simulink model "AW_PMSMwTorqueRipple"  (R2021b)
settings: Solver=VariableStepAuto  StartTime=0.0  StopTime=100  MaxStep=ts  RelTol=1e-3
values from neighbouring files (symbols this model uses):
  alfa = atan(sqrt(3)*dia / (dia + 2*dib))    [AW_RippleModel_InitFcn.m]
  delta_T = diqA*K_t    [AW_RippleModel_InitFcn.m]
  Jz = 0.753    [AW_RippleModel_InitFcn.m]
  K_t = 17.5    [AW_RippleModel_InitFcn.m]
  p = 24    [AW_RippleModel_InitFcn.m]
  PID_GA_b = 1    [AW_RippleModel_InitFcn.m]
  PID_GA_Kd = 4.772*(88.300/1000)    (= 0.4213676)    [AW_RippleModel_InitFcn.m]
  PID_GA_Ki = 4.772/(0.153/1000)    (= 31189.5424837)    [AW_RippleModel_InitFcn.m]
  PID_GA_Kp = 4.772    [AW_RippleModel_InitFcn.m]
  PID_Ki = Jz  * ((2*pi*fref)^2)    (= 2972.72484561)    [AW_RippleModel_InitFcn.m]
  PID_Kp = (2*eref*Jz) * (2*pi*fref)    (= 85.1622936535)    [AW_RippleModel_InitFcn.m]
  Tn = 50    [AW_RippleModel_InitFcn.m]
libraries: slpidlib x7, cstblocks x4, simulink x1, fuzblock x1
settings Model: Creator=AW  LastModifiedBy=adria
settings SolverCC: AlgebraicLoopSolver=TrustRegion  PositivePriorityOrder=on
settings DataIOCC: ReturnWorkspaceOutputs=off
settings DebuggingCC: SFMachineParentedDataDiag=warning  ArithmeticOperatorsInVariantConditions=warning
settings SFSimCC: SimUseLocalCustomCode=off  CustomCodeUndefinedFunction=UseInterfaceOnly
settings RTWCC: RTWUseLocalCustomCode=off

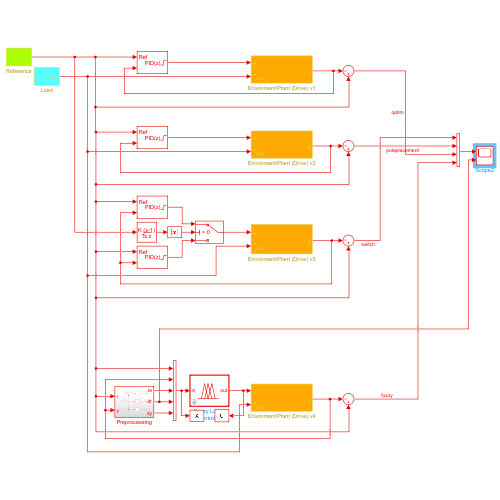
[thumbnail: Simulink's stored preview of the top-level diagram]
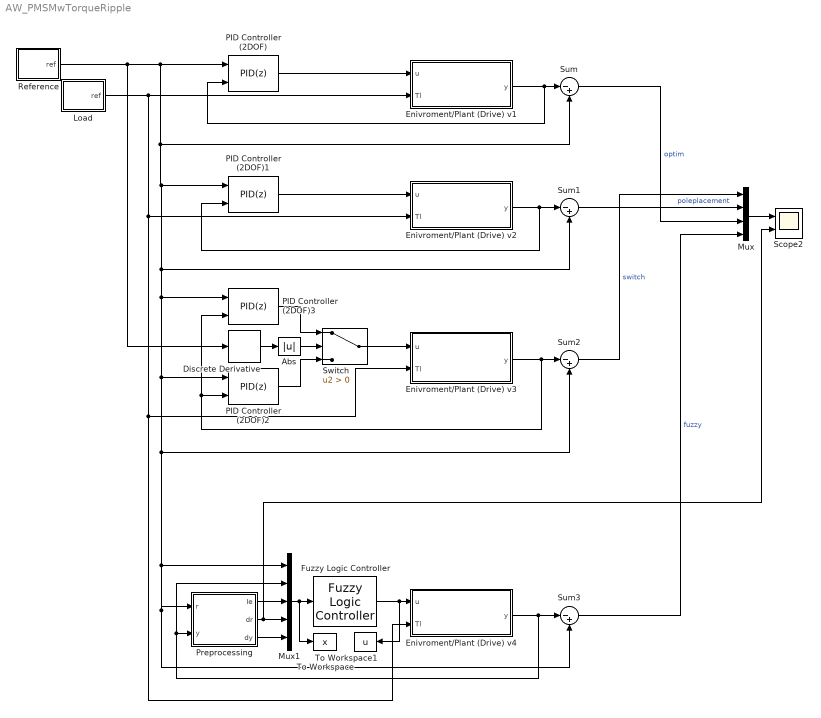
== system AW_PMSMwTorqueRipple ==
  Abs : Abs
  Discrete Derivative : simulink/Quick Insert/Discrete/Discrete Derivative  gainval=1.0  ICPrevScaledInput=0.0  OutMin=[]  OutMax=[]  OutDataType=fixdt(1, 16)  OutScaling=2^-10  DoSatur=off
      settings: SourceProductBaseCode=SL
  Enivroment/Plant (Drive) v1 : Subsystem
      mask Display:
      | port_label('input', 1, 'u', 'texmode', 'on')
      | port_label('input', 2, 'T_{load}', 'texmode', 'on')
      | port_label('output', 1, 'y', 'texmode', 'on')
  Enivroment/Plant (Drive) v2 : Subsystem
      mask Display:
      | port_label('input', 1, 'u', 'texmode', 'on')
      | port_label('input', 2, 'T_{load}', 'texmode', 'on')
      | port_label('output', 1, 'y', 'texmode', 'on')
  Enivroment/Plant (Drive) v3 : Subsystem
      mask Display:
      | port_label('input', 1, 'u', 'texmode', 'on')
      | port_label('input', 2, 'T_{load}', 'texmode', 'on')
      | port_label('output', 1, 'y', 'texmode', 'on')
  Enivroment/Plant (Drive) v4 : Subsystem
      mask Display:
      | port_label('input', 1, 'u', 'texmode', 'on')
      | port_label('input', 2, 'T_{load}', 'texmode', 'on')
      | port_label('output', 1, 'y', 'texmode', 'on')
  Fuzzy Logic Controller : fuzblock/Fuzzy Logic  Controller  FIS=PMSM_SpeedController  OutputSampleNumber=101  DataType=double  FuzzifiedInputs=off  RuleFiringStrengths=off  RuleOutputs=off  AggregatedOutputs=off  SimulateUsing=Code generation  OutOfRangeInputValueMessage=warning  NoRuleFiredMessage=warning  EmptyOutputFuzzySetMessage=warning
  Load : Subsystem
      mask Display: port_label('output', 1, 'T_{load}', 'texmode', 'on')
  Mux : Mux
  Mux1 : Mux  Inputs=5
  PID Controller (2DOF) : slpidlib/PID Controller (2DOF)  Controller=PID  Form=Parallel  TimeDomain=Discrete-time  UseExternalTs=off  SampleTime=-1  IntegratorMethod=Forward Euler  FilterMethod=Forward Euler  ControllerParametersSource=internal  P=PID_GA_Kp  I=PID_GA_Ki  D=PID_GA_Kd  UseFilter=on  N=100  b=PID_GA_b  c=PID_GA_c  TunerSelectOption=Transfer Function Based (PID Tuner App)  InitialConditionSource=internal  InitialConditionForIntegrator=0  InitialConditionForFilter=0  DifferentiatorICPrevScaledInput=0  ExternalReset=none  TrackingMode=off  Kt=1  LimitOutput=on  SatLimitsSource=internal  UpperSaturationLimit=6  LowerSaturationLimit=-6  LinearizeAsGain=on  AntiWindupMode=none  Kb=1  POutMin=[]  POutMax=[]  IOutMin=[]  IOutMax=[]  DOutMin=[]  DOutMax=[]  NOutMin=[]  NOutMax=[]  bOutMin=[]  bOutMax=[]  cOutMin=[]  cOutMax=[]  SumOutMin=[]  SumOutMax=[]  SaturationOutMin=[]  SaturationOutMax=[]  PParamMin=[]  PParamMax=[]  IParamMin=[]  IParamMax=[]  DParamMin=[]  DParamMax=[]  NParamMin=[]  NParamMax=[]  bParamMin=[]  bParamMax=[]  cParamMin=[]  cParamMax=[]  KbParamMin=[]  KbParamMax=[]  KtParamMin=[]  KtParamMax=[]  KbOutMin=[]  KbOutMax=[]  KtOutMin=[]  KtOutMax=[]  IntegratorOutMin=[]  IntegratorOutMax=[]  FilterOutMin=[]  FilterOutMax=[]  SumI1OutMin=[]  SumI1OutMax=[]  SumI2OutMin=[]  SumI2OutMax=[]  SumI3OutMin=[]  SumI3OutMax=[]  SumI4OutMin=[]  SumI4OutMax=[]  SumDOutMin=[]  SumDOutMax=[]  Sum1OutMin=[]  Sum1OutMax=[]  Sum2OutMin=[]  Sum2OutMax=[]  Sum3OutMin=[]  Sum3OutMax=[]  DifferentiatorOutMin=[]  DifferentiatorOutMax=[]  FilterDiffOutCoefMin=[]  FilterDiffOutCoefMax=[]  ReciprocalOutMin=[]  ReciprocalOutMax=[]  SumDenOutMin=[]  SumDenOutMax=[]  SumNumOutMin=[]  SumNumOutMax=[]  DivideOutMin=[]  DivideOutMax=[]  UdiffTsProdOutMin=[]  UdiffTsProdOutMax=[]  NTsProdOutMin=[]  NTsProdOutMax=[]  UintegralTsProdOutMin=[]  UintegralTsProdOutMax=[]  UngainTsProdOutMin=[]  UngainTsProdOutMax=[]  IntegratorContinuousStateAttributes=''  IntegratorStateMustResolveToSignalObject=off  IntegratorRTWStateStorageClass=Auto  FilterContinuousStateAttributes=''  FilterStateMustResolveToSignalObject=off  FilterRTWStateStorageClass=Auto  ParallelPVariant=InternalParameters  IdealPVariant=Disabled  IVariant=InternalParameters  DVariant=InternalParameters  bVariant=InternalParameters  cVariant=InternalParameters  IntegratorVariant=Discrete  SatVariant=Enabled  AWVariant=Passthrough  PCopyVariant=Disabled  TRVariant=Disabled  FdbkBlocksVariant=Forward  IdealPFdbkVariant=Disabled  SatFdbkVariant=Disabled  DerivativeFilterVariant=ForwardEulerFilter  NVariant=InternalParameters  NCopyVariant=Disabled  FilterICVariant=InternalICsFilter  IntegratorICVariant=InternalICs  ExternalResetVariant=Disabled  TRSumVariant=Passthrough  SumFdbkVariant=Disabled  SumVariant=Sum_PID  TsampFilterVariant=InternalTs  TsampNgainVariant=Passthrough  TsampIntegralVariant=Passthrough  ExternalSaturationOutDataTypeStr=Inherit: Same as second input
      settings: SourceProductBaseCode=SL
  PID Controller (2DOF)1 : slpidlib/PID Controller (2DOF)  Controller=PID  Form=Parallel  TimeDomain=Discrete-time  UseExternalTs=off  SampleTime=-1  IntegratorMethod=Forward Euler  FilterMethod=Forward Euler  ControllerParametersSource=internal  P=PID_Kp  I=PID_Ki  D=0  UseFilter=on  N=100  b=1  c=0  TunerSelectOption=Transfer Function Based (PID Tuner App)  InitialConditionSource=internal  InitialConditionForIntegrator=0  InitialConditionForFilter=0  DifferentiatorICPrevScaledInput=0  ExternalReset=none  TrackingMode=off  Kt=1  LimitOutput=on  SatLimitsSource=internal  UpperSaturationLimit=6  LowerSaturationLimit=-6  LinearizeAsGain=on  AntiWindupMode=none  Kb=1  POutMin=[]  POutMax=[]  IOutMin=[]  IOutMax=[]  DOutMin=[]  DOutMax=[]  NOutMin=[]  NOutMax=[]  bOutMin=[]  bOutMax=[]  cOutMin=[]  cOutMax=[]  SumOutMin=[]  SumOutMax=[]  SaturationOutMin=[]  SaturationOutMax=[]  PParamMin=[]  PParamMax=[]  IParamMin=[]  IParamMax=[]  DParamMin=[]  DParamMax=[]  NParamMin=[]  NParamMax=[]  bParamMin=[]  bParamMax=[]  cParamMin=[]  cParamMax=[]  KbParamMin=[]  KbParamMax=[]  KtParamMin=[]  KtParamMax=[]  KbOutMin=[]  KbOutMax=[]  KtOutMin=[]  KtOutMax=[]  IntegratorOutMin=[]  IntegratorOutMax=[]  FilterOutMin=[]  FilterOutMax=[]  SumI1OutMin=[]  SumI1OutMax=[]  SumI2OutMin=[]  SumI2OutMax=[]  SumI3OutMin=[]  SumI3OutMax=[]  SumI4OutMin=[]  SumI4OutMax=[]  SumDOutMin=[]  SumDOutMax=[]  Sum1OutMin=[]  Sum1OutMax=[]  Sum2OutMin=[]  Sum2OutMax=[]  Sum3OutMin=[]  Sum3OutMax=[]  DifferentiatorOutMin=[]  DifferentiatorOutMax=[]  FilterDiffOutCoefMin=[]  FilterDiffOutCoefMax=[]  ReciprocalOutMin=[]  ReciprocalOutMax=[]  SumDenOutMin=[]  SumDenOutMax=[]  SumNumOutMin=[]  SumNumOutMax=[]  DivideOutMin=[]  DivideOutMax=[]  UdiffTsProdOutMin=[]  UdiffTsProdOutMax=[]  NTsProdOutMin=[]  NTsProdOutMax=[]  UintegralTsProdOutMin=[]  UintegralTsProdOutMax=[]  UngainTsProdOutMin=[]  UngainTsProdOutMax=[]  IntegratorContinuousStateAttributes=''  IntegratorStateMustResolveToSignalObject=off  IntegratorRTWStateStorageClass=Auto  FilterContinuousStateAttributes=''  FilterStateMustResolveToSignalObject=off  FilterRTWStateStorageClass=Auto  ParallelPVariant=InternalParameters  IdealPVariant=Disabled  IVariant=InternalParameters  DVariant=InternalParameters  bVariant=InternalParameters  cVariant=InternalParameters  IntegratorVariant=Discrete  SatVariant=Enabled  AWVariant=Passthrough  PCopyVariant=Disabled  TRVariant=Disabled  FdbkBlocksVariant=Forward  IdealPFdbkVariant=Disabled  SatFdbkVariant=Disabled  DerivativeFilterVariant=ForwardEulerFilter  NVariant=InternalParameters  NCopyVariant=Disabled  FilterICVariant=InternalICsFilter  IntegratorICVariant=InternalICs  ExternalResetVariant=Disabled  TRSumVariant=Passthrough  SumFdbkVariant=Disabled  SumVariant=Sum_PID  TsampFilterVariant=InternalTs  TsampNgainVariant=Passthrough  TsampIntegralVariant=Passthrough  ExternalSaturationOutDataTypeStr=Inherit: Same as second input
      settings: SourceProductBaseCode=SL
  PID Controller (2DOF)2 : slpidlib/PID Controller (2DOF)  Controller=PID  Form=Parallel  TimeDomain=Discrete-time  UseExternalTs=off  SampleTime=-1  IntegratorMethod=Forward Euler  FilterMethod=Forward Euler  ControllerParametersSource=internal  P=4.772  I=4.772/(0.153/1000)  D=4.772*(88.300/1000)  UseFilter=on  N=100  b=1  c=0.258  TunerSelectOption=Transfer Function Based (PID Tuner App)  InitialConditionSource=internal  InitialConditionForIntegrator=0  InitialConditionForFilter=0  DifferentiatorICPrevScaledInput=0  ExternalReset=none  TrackingMode=off  Kt=1  LimitOutput=on  SatLimitsSource=internal  UpperSaturationLimit=6  LowerSaturationLimit=-6  LinearizeAsGain=on  AntiWindupMode=none  Kb=1  POutMin=[]  POutMax=[]  IOutMin=[]  IOutMax=[]  DOutMin=[]  DOutMax=[]  NOutMin=[]  NOutMax=[]  bOutMin=[]  bOutMax=[]  cOutMin=[]  cOutMax=[]  SumOutMin=[]  SumOutMax=[]  SaturationOutMin=[]  SaturationOutMax=[]  PParamMin=[]  PParamMax=[]  IParamMin=[]  IParamMax=[]  DParamMin=[]  DParamMax=[]  NParamMin=[]  NParamMax=[]  bParamMin=[]  bParamMax=[]  cParamMin=[]  cParamMax=[]  KbParamMin=[]  KbParamMax=[]  KtParamMin=[]  KtParamMax=[]  KbOutMin=[]  KbOutMax=[]  KtOutMin=[]  KtOutMax=[]  IntegratorOutMin=[]  IntegratorOutMax=[]  FilterOutMin=[]  FilterOutMax=[]  SumI1OutMin=[]  SumI1OutMax=[]  SumI2OutMin=[]  SumI2OutMax=[]  SumI3OutMin=[]  SumI3OutMax=[]  SumI4OutMin=[]  SumI4OutMax=[]  SumDOutMin=[]  SumDOutMax=[]  Sum1OutMin=[]  Sum1OutMax=[]  Sum2OutMin=[]  Sum2OutMax=[]  Sum3OutMin=[]  Sum3OutMax=[]  DifferentiatorOutMin=[]  DifferentiatorOutMax=[]  FilterDiffOutCoefMin=[]  FilterDiffOutCoefMax=[]  ReciprocalOutMin=[]  ReciprocalOutMax=[]  SumDenOutMin=[]  SumDenOutMax=[]  SumNumOutMin=[]  SumNumOutMax=[]  DivideOutMin=[]  DivideOutMax=[]  UdiffTsProdOutMin=[]  UdiffTsProdOutMax=[]  NTsProdOutMin=[]  NTsProdOutMax=[]  UintegralTsProdOutMin=[]  UintegralTsProdOutMax=[]  UngainTsProdOutMin=[]  UngainTsProdOutMax=[]  IntegratorContinuousStateAttributes=''  IntegratorStateMustResolveToSignalObject=off  IntegratorRTWStateStorageClass=Auto  FilterContinuousStateAttributes=''  FilterStateMustResolveToSignalObject=off  FilterRTWStateStorageClass=Auto  ParallelPVariant=InternalParameters  IdealPVariant=Disabled  IVariant=InternalParameters  DVariant=InternalParameters  bVariant=InternalParameters  cVariant=InternalParameters  IntegratorVariant=Discrete  SatVariant=Enabled  AWVariant=Passthrough  PCopyVariant=Disabled  TRVariant=Disabled  FdbkBlocksVariant=Forward  IdealPFdbkVariant=Disabled  SatFdbkVariant=Disabled  DerivativeFilterVariant=ForwardEulerFilter  NVariant=InternalParameters  NCopyVariant=Disabled  FilterICVariant=InternalICsFilter  IntegratorICVariant=InternalICs  ExternalResetVariant=Disabled  TRSumVariant=Passthrough  SumFdbkVariant=Disabled  SumVariant=Sum_PID  TsampFilterVariant=InternalTs  TsampNgainVariant=Passthrough  TsampIntegralVariant=Passthrough  ExternalSaturationOutDataTypeStr=Inherit: Same as second input
      settings: SourceProductBaseCode=SL
  PID Controller (2DOF)3 : slpidlib/PID Controller (2DOF)  Controller=PID  Form=Parallel  TimeDomain=Discrete-time  UseExternalTs=off  SampleTime=-1  IntegratorMethod=Forward Euler  FilterMethod=Forward Euler  ControllerParametersSource=internal  P=PID_Kp  I=PID_Ki  D=0  UseFilter=on  N=100  b=1  c=0  TunerSelectOption=Transfer Function Based (PID Tuner App)  InitialConditionSource=internal  InitialConditionForIntegrator=0  InitialConditionForFilter=0  DifferentiatorICPrevScaledInput=0  ExternalReset=none  TrackingMode=off  Kt=1  LimitOutput=on  SatLimitsSource=internal  UpperSaturationLimit=6  LowerSaturationLimit=-6  LinearizeAsGain=on  AntiWindupMode=none  Kb=1  POutMin=[]  POutMax=[]  IOutMin=[]  IOutMax=[]  DOutMin=[]  DOutMax=[]  NOutMin=[]  NOutMax=[]  bOutMin=[]  bOutMax=[]  cOutMin=[]  cOutMax=[]  SumOutMin=[]  SumOutMax=[]  SaturationOutMin=[]  SaturationOutMax=[]  PParamMin=[]  PParamMax=[]  IParamMin=[]  IParamMax=[]  DParamMin=[]  DParamMax=[]  NParamMin=[]  NParamMax=[]  bParamMin=[]  bParamMax=[]  cParamMin=[]  cParamMax=[]  KbParamMin=[]  KbParamMax=[]  KtParamMin=[]  KtParamMax=[]  KbOutMin=[]  KbOutMax=[]  KtOutMin=[]  KtOutMax=[]  IntegratorOutMin=[]  IntegratorOutMax=[]  FilterOutMin=[]  FilterOutMax=[]  SumI1OutMin=[]  SumI1OutMax=[]  SumI2OutMin=[]  SumI2OutMax=[]  SumI3OutMin=[]  SumI3OutMax=[]  SumI4OutMin=[]  SumI4OutMax=[]  SumDOutMin=[]  SumDOutMax=[]  Sum1OutMin=[]  Sum1OutMax=[]  Sum2OutMin=[]  Sum2OutMax=[]  Sum3OutMin=[]  Sum3OutMax=[]  DifferentiatorOutMin=[]  DifferentiatorOutMax=[]  FilterDiffOutCoefMin=[]  FilterDiffOutCoefMax=[]  ReciprocalOutMin=[]  ReciprocalOutMax=[]  SumDenOutMin=[]  SumDenOutMax=[]  SumNumOutMin=[]  SumNumOutMax=[]  DivideOutMin=[]  DivideOutMax=[]  UdiffTsProdOutMin=[]  UdiffTsProdOutMax=[]  NTsProdOutMin=[]  NTsProdOutMax=[]  UintegralTsProdOutMin=[]  UintegralTsProdOutMax=[]  UngainTsProdOutMin=[]  UngainTsProdOutMax=[]  IntegratorContinuousStateAttributes=''  IntegratorStateMustResolveToSignalObject=off  IntegratorRTWStateStorageClass=Auto  FilterContinuousStateAttributes=''  FilterStateMustResolveToSignalObject=off  FilterRTWStateStorageClass=Auto  ParallelPVariant=InternalParameters  IdealPVariant=Disabled  IVariant=InternalParameters  DVariant=InternalParameters  bVariant=InternalParameters  cVariant=InternalParameters  IntegratorVariant=Discrete  SatVariant=Enabled  AWVariant=Passthrough  PCopyVariant=Disabled  TRVariant=Disabled  FdbkBlocksVariant=Forward  IdealPFdbkVariant=Disabled  SatFdbkVariant=Disabled  DerivativeFilterVariant=ForwardEulerFilter  NVariant=InternalParameters  NCopyVariant=Disabled  FilterICVariant=InternalICsFilter  IntegratorICVariant=InternalICs  ExternalResetVariant=Disabled  TRSumVariant=Passthrough  SumFdbkVariant=Disabled  SumVariant=Sum_PID  TsampFilterVariant=InternalTs  TsampNgainVariant=Passthrough  TsampIntegralVariant=Passthrough  ExternalSaturationOutDataTypeStr=Inherit: Same as second input
      settings: SourceProductBaseCode=SL
  Preprocessing : Subsystem
  Reference : Subsystem
      mask Display: port_label('output', 1, 'y_{ref}', 'texmode', 'on')
  Scope2 : Scope  NumInputPorts=2
  Sum{,1..3} (4 alike) : Sum  Inputs=|-+
  Switch : Switch  Criteria=u2 > Threshold
  To Workspace : ToWorkspace  VariableName=x  SaveFormat=Timeseries  SampleTime=-1
  To Workspace1 : ToWorkspace  VariableName=u  SaveFormat=Timeseries  SampleTime=-1
  wires:
  Sum/1 -> Mux/3  "optim"
  Sum1/1 -> Mux/2  "poleplacement"
  Load/1(ref) -> Enivroment/Plant (Drive) v2/2(Tl), Enivroment/Plant (Drive) v4/2(Tl), Enivroment/Plant (Drive) v3/2(Tl), Enivroment/Plant (Drive) v1/2(Tl)
  Enivroment/Plant (Drive) v2/1(y) -> Sum1/1, PID Controller (2DOF)1/2
  PID Controller (2DOF)1/1 -> Enivroment/Plant (Drive) v2/1(u)
  Mux/1 -> Scope2/1
  Discrete Derivative/1 -> Abs/1
  Abs/1 -> Switch/2
  PID Controller (2DOF)3/1 -> Switch/1
  Switch/1 -> Enivroment/Plant (Drive) v3/1(u)
  Enivroment/Plant (Drive) v3/1(y) -> Sum2/1, PID Controller (2DOF)3/2, PID Controller (2DOF)2/2
  Sum2/1 -> Mux/1  "switch"
  PID Controller (2DOF)2/1 -> Switch/3
  Preprocessing/3(dy) -> Mux1/5
  Preprocessing/2(dr) -> Scope2/2, Mux1/4
  Preprocessing/1(Ie) -> Mux1/3
  Mux1/1 -> To Workspace/1, Fuzzy Logic Controller/1
  Fuzzy Logic Controller/1 -> To Workspace1/1, Enivroment/Plant (Drive) v4/1(u)
  Enivroment/Plant (Drive) v4/1(y) -> Sum3/1, Preprocessing/2(y), Mux1/2
  PID Controller (2DOF)/1 -> Enivroment/Plant (Drive) v1/1(u)
  Sum3/1 -> Mux/4  "fuzzy"
  Enivroment/Plant (Drive) v1/1(y) -> Sum/1, PID Controller (2DOF)/2
  Reference/1(ref) -> Discrete Derivative/1, Sum/2, Sum1/2, Sum2/2, Mux1/1, Preprocessing/1(r), Sum3/2, PID Controller (2DOF)2/1, PID Controller (2DOF)3/1, PID Controller (2DOF)1/1, PID Controller (2DOF)/1

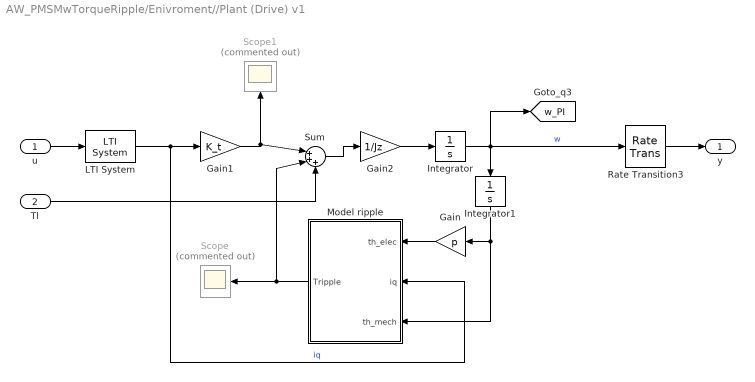
== system AW_PMSMwTorqueRipple/Enivroment//Plant (Drive) v1 ==
  u : Inport
  Tl : Inport  Port=2
  Gain : Gain  Gain=p
  Gain1 : Gain  Gain=K_t
  Gain2 : Gain  Gain=1/Jz
  Integrator : Integrator
  Integrator1 : Integrator
  LTI System : cstblocks/LTI System  sys=h_curr  IC=[]
  Model ripple : Subsystem
  Rate Transition3 : RateTransition  OutPortSampleTime=ts
  Scope : Scope  Commented=on
  Scope1 : Scope  Commented=on
  Sum : Sum  Inputs=|+++
  y : Outport  VectorParamsAs1DForOutWhenUnconnected=off
  tag scope: w_PI=global
  wires:
  Gain/1 -> Model ripple/1(th_elec)
  Integrator/1 -> [w_PI], Rate Transition3/1, Integrator1/1  "w"
  u/1 -> LTI System/1
  Gain2/1 -> Integrator/1
  Sum/1 -> Gain2/1
  Model ripple/1(Tripple) -> Sum/2, Scope/1
  Gain1/1 -> Scope1/1, Sum/1
  Integrator1/1 -> Model ripple/3(th_mech), Gain/1
  LTI System/1 -> Gain1/1, Model ripple/2(iq)  "iq"
  Tl/1 -> Sum/3
  Rate Transition3/1 -> y/1

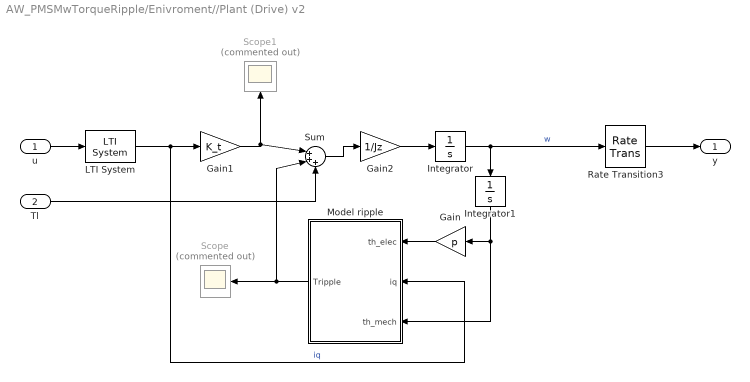
== system AW_PMSMwTorqueRipple/Enivroment//Plant (Drive) v2 ==
  u : Inport
  Tl : Inport  Port=2
  Gain : Gain  Gain=p
  Gain1 : Gain  Gain=K_t
  Gain2 : Gain  Gain=1/Jz
  Integrator : Integrator
  Integrator1 : Integrator
  LTI System : cstblocks/LTI System  sys=h_curr  IC=[]
  Model ripple : Subsystem
  Rate Transition3 : RateTransition  OutPortSampleTime=ts
  Scope : Scope  Commented=on
  Scope1 : Scope  Commented=on
  Sum : Sum  Inputs=|+++
  y : Outport  VectorParamsAs1DForOutWhenUnconnected=off
  wires:
  Gain/1 -> Model ripple/1(th_elec)
  Integrator/1 -> Rate Transition3/1, Integrator1/1  "w"
  u/1 -> LTI System/1
  Gain2/1 -> Integrator/1
  Sum/1 -> Gain2/1
  Model ripple/1(Tripple) -> Sum/2, Scope/1
  Gain1/1 -> Scope1/1, Sum/1
  Integrator1/1 -> Model ripple/3(th_mech), Gain/1
  LTI System/1 -> Gain1/1, Model ripple/2(iq)  "iq"
  Tl/1 -> Sum/3
  Rate Transition3/1 -> y/1

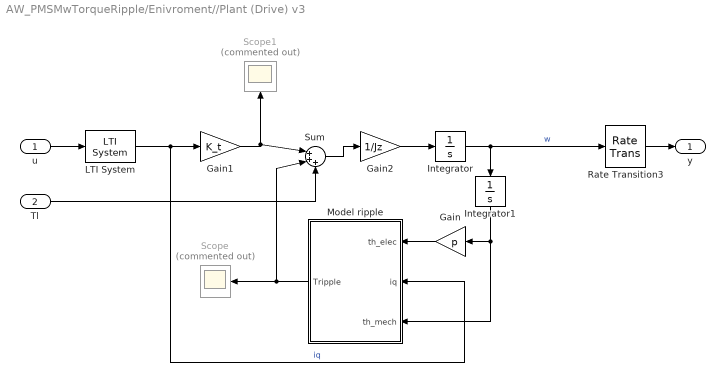
== system AW_PMSMwTorqueRipple/Enivroment//Plant (Drive) v3 ==
  u : Inport
  Tl : Inport  Port=2
  Gain : Gain  Gain=p
  Gain1 : Gain  Gain=K_t
  Gain2 : Gain  Gain=1/Jz
  Integrator : Integrator
  Integrator1 : Integrator
  LTI System : cstblocks/LTI System  sys=h_curr  IC=[]
  Model ripple : Subsystem
  Rate Transition3 : RateTransition  OutPortSampleTime=ts
  Scope : Scope  Commented=on
  Scope1 : Scope  Commented=on
  Sum : Sum  Inputs=|+++
  y : Outport  VectorParamsAs1DForOutWhenUnconnected=off
  wires:
  Gain/1 -> Model ripple/1(th_elec)
  Integrator/1 -> Rate Transition3/1, Integrator1/1  "w"
  u/1 -> LTI System/1
  Gain2/1 -> Integrator/1
  Sum/1 -> Gain2/1
  Model ripple/1(Tripple) -> Sum/2, Scope/1
  Gain1/1 -> Scope1/1, Sum/1
  Integrator1/1 -> Model ripple/3(th_mech), Gain/1
  LTI System/1 -> Gain1/1, Model ripple/2(iq)  "iq"
  Tl/1 -> Sum/3
  Rate Transition3/1 -> y/1

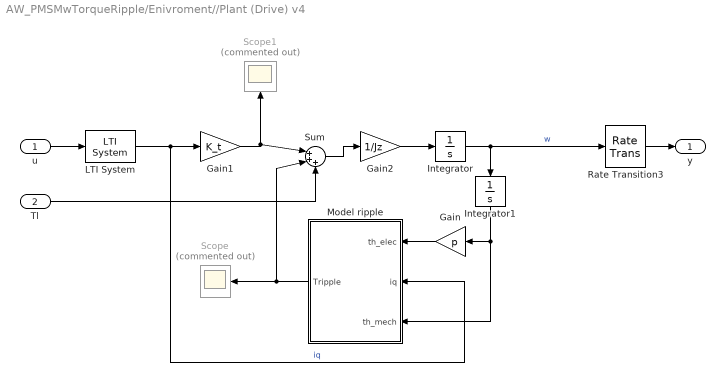
== system AW_PMSMwTorqueRipple/Enivroment//Plant (Drive) v4 ==
  u : Inport
  Tl : Inport  Port=2
  Gain : Gain  Gain=p
  Gain1 : Gain  Gain=K_t
  Gain2 : Gain  Gain=1/Jz
  Integrator : Integrator
  Integrator1 : Integrator
  LTI System : cstblocks/LTI System  sys=h_curr  IC=[]
  Model ripple : Subsystem
  Rate Transition3 : RateTransition  OutPortSampleTime=ts
  Scope : Scope  Commented=on
  Scope1 : Scope  Commented=on
  Sum : Sum  Inputs=|+++
  y : Outport  VectorParamsAs1DForOutWhenUnconnected=off
  wires:
  Gain/1 -> Model ripple/1(th_elec)
  Integrator/1 -> Rate Transition3/1, Integrator1/1  "w"
  u/1 -> LTI System/1
  Gain2/1 -> Integrator/1
  Sum/1 -> Gain2/1
  Model ripple/1(Tripple) -> Sum/2, Scope/1
  Gain1/1 -> Scope1/1, Sum/1
  Integrator1/1 -> Model ripple/3(th_mech), Gain/1
  LTI System/1 -> Gain1/1, Model ripple/2(iq)  "iq"
  Tl/1 -> Sum/3
  Rate Transition3/1 -> y/1

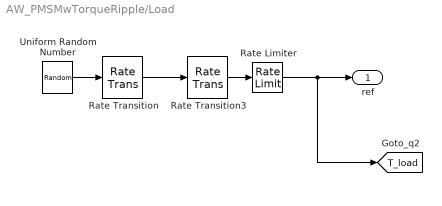
== system AW_PMSMwTorqueRipple/Load ==
  Rate Limiter : RateLimiter  RisingSlewLimit=50/0.1  FallingSlewLimit=-50/0.1  SampleTimeMode=inherited
  Rate Transition : RateTransition
  Rate Transition3 : RateTransition  OutPortSampleTime=ts
  Uniform Random Number : UniformRandomNumber  Minimum=-50  Maximum=50  Seed=321  SampleTime=100
  ref : Outport  VectorParamsAs1DForOutWhenUnconnected=off
  tag scope: T_load=global
  wires:
  Rate Transition/1 -> Rate Transition3/1
  Uniform Random Number/1 -> Rate Transition/1
  Rate Transition3/1 -> Rate Limiter/1
  Rate Limiter/1 -> [T_load], ref/1

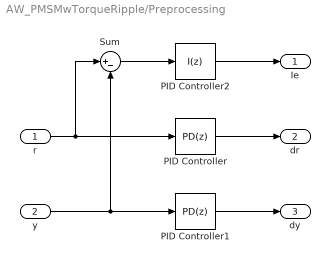
== system AW_PMSMwTorqueRipple/Preprocessing ==
  r : Inport
  y : Inport  Port=2
  PID Controller : slpidlib/PID Controller  Controller=PD  Form=Parallel  TimeDomain=Discrete-time  UseExternalTs=off  SampleTime=-1  IntegratorMethod=Forward Euler  FilterMethod=Forward Euler  ControllerParametersSource=internal  P=0  I=1  D=1  UseFilter=on  N=10  TunerSelectOption=Transfer Function Based (PID Tuner App)  InitialConditionSource=internal  InitialConditionForIntegrator=0  InitialConditionForFilter=0  DifferentiatorICPrevScaledInput=0  ExternalReset=none  TrackingMode=off  Kt=1  LimitOutput=off  SatLimitsSource=internal  UpperSaturationLimit=inf  LowerSaturationLimit=-inf  LinearizeAsGain=on  AntiWindupMode=none  Kb=1  POutMin=[]  POutMax=[]  IOutMin=[]  IOutMax=[]  DOutMin=[]  DOutMax=[]  NOutMin=[]  NOutMax=[]  SumOutMin=[]  SumOutMax=[]  SaturationOutMin=[]  SaturationOutMax=[]  PParamMin=[]  PParamMax=[]  IParamMin=[]  IParamMax=[]  DParamMin=[]  DParamMax=[]  NParamMin=[]  NParamMax=[]  KbParamMin=[]  KbParamMax=[]  KtParamMin=[]  KtParamMax=[]  KbOutMin=[]  KbOutMax=[]  KtOutMin=[]  KtOutMax=[]  IntegratorOutMin=[]  IntegratorOutMax=[]  FilterOutMin=[]  FilterOutMax=[]  SumI1OutMin=[]  SumI1OutMax=[]  SumI2OutMin=[]  SumI2OutMax=[]  SumI3OutMin=[]  SumI3OutMax=[]  SumI4OutMin=[]  SumI4OutMax=[]  SumDOutMin=[]  SumDOutMax=[]  DifferentiatorOutMin=[]  DifferentiatorOutMax=[]  FilterDiffOutCoefMin=[]  FilterDiffOutCoefMax=[]  ReciprocalOutMin=[]  ReciprocalOutMax=[]  SumDenOutMin=[]  SumDenOutMax=[]  SumNumOutMin=[]  SumNumOutMax=[]  DivideOutMin=[]  DivideOutMax=[]  UdiffTsProdOutMin=[]  UdiffTsProdOutMax=[]  NTsProdOutMin=[]  NTsProdOutMax=[]  UintegralTsProdOutMin=[]  UintegralTsProdOutMax=[]  UngainTsProdOutMin=[]  UngainTsProdOutMax=[]  IntegratorContinuousStateAttributes=''  IntegratorStateMustResolveToSignalObject=off  IntegratorRTWStateStorageClass=Auto  FilterContinuousStateAttributes=''  FilterStateMustResolveToSignalObject=off  FilterRTWStateStorageClass=Auto  ParallelPVariant=InternalParameters  IdealPVariant=Disabled  IVariant=Disabled  DVariant=InternalParameters  IntegratorVariant=Disabled  SatVariant=Disabled  AWVariant=Disabled  PCopyVariant=Disabled  TRVariant=Disabled  FdbkBlocksVariant=Forward  IdealPFdbkVariant=Disabled  SatFdbkVariant=Disabled  DerivativeFilterVariant=ForwardEulerFilter  NVariant=InternalParameters  NCopyVariant=Disabled  FilterICVariant=InternalICsFilter  IntegratorICVariant=Disabled  ExternalResetVariant=Disabled  TRSumVariant=Passthrough  SumFdbkVariant=Disabled  SumVariant=Sum_PD  TsampFilterVariant=InternalTs  TsampNgainVariant=Passthrough  TsampIntegralVariant=Disabled_SignalSpec  ExternalSaturationOutDataTypeStr=Inherit: Same as second input
  PID Controller1 : slpidlib/PID Controller  Controller=PD  Form=Parallel  TimeDomain=Discrete-time  UseExternalTs=off  SampleTime=-1  IntegratorMethod=Forward Euler  FilterMethod=Forward Euler  ControllerParametersSource=internal  P=0  I=1  D=1  UseFilter=on  N=100  TunerSelectOption=Transfer Function Based (PID Tuner App)  InitialConditionSource=internal  InitialConditionForIntegrator=0  InitialConditionForFilter=0  DifferentiatorICPrevScaledInput=0  ExternalReset=none  TrackingMode=off  Kt=1  LimitOutput=off  SatLimitsSource=internal  UpperSaturationLimit=inf  LowerSaturationLimit=-inf  LinearizeAsGain=on  AntiWindupMode=none  Kb=1  POutMin=[]  POutMax=[]  IOutMin=[]  IOutMax=[]  DOutMin=[]  DOutMax=[]  NOutMin=[]  NOutMax=[]  SumOutMin=[]  SumOutMax=[]  SaturationOutMin=[]  SaturationOutMax=[]  PParamMin=[]  PParamMax=[]  IParamMin=[]  IParamMax=[]  DParamMin=[]  DParamMax=[]  NParamMin=[]  NParamMax=[]  KbParamMin=[]  KbParamMax=[]  KtParamMin=[]  KtParamMax=[]  KbOutMin=[]  KbOutMax=[]  KtOutMin=[]  KtOutMax=[]  IntegratorOutMin=[]  IntegratorOutMax=[]  FilterOutMin=[]  FilterOutMax=[]  SumI1OutMin=[]  SumI1OutMax=[]  SumI2OutMin=[]  SumI2OutMax=[]  SumI3OutMin=[]  SumI3OutMax=[]  SumI4OutMin=[]  SumI4OutMax=[]  SumDOutMin=[]  SumDOutMax=[]  DifferentiatorOutMin=[]  DifferentiatorOutMax=[]  FilterDiffOutCoefMin=[]  FilterDiffOutCoefMax=[]  ReciprocalOutMin=[]  ReciprocalOutMax=[]  SumDenOutMin=[]  SumDenOutMax=[]  SumNumOutMin=[]  SumNumOutMax=[]  DivideOutMin=[]  DivideOutMax=[]  UdiffTsProdOutMin=[]  UdiffTsProdOutMax=[]  NTsProdOutMin=[]  NTsProdOutMax=[]  UintegralTsProdOutMin=[]  UintegralTsProdOutMax=[]  UngainTsProdOutMin=[]  UngainTsProdOutMax=[]  IntegratorContinuousStateAttributes=''  IntegratorStateMustResolveToSignalObject=off  IntegratorRTWStateStorageClass=Auto  FilterContinuousStateAttributes=''  FilterStateMustResolveToSignalObject=off  FilterRTWStateStorageClass=Auto  ParallelPVariant=InternalParameters  IdealPVariant=Disabled  IVariant=Disabled  DVariant=InternalParameters  IntegratorVariant=Disabled  SatVariant=Disabled  AWVariant=Disabled  PCopyVariant=Disabled  TRVariant=Disabled  FdbkBlocksVariant=Forward  IdealPFdbkVariant=Disabled  SatFdbkVariant=Disabled  DerivativeFilterVariant=ForwardEulerFilter  NVariant=InternalParameters  NCopyVariant=Disabled  FilterICVariant=InternalICsFilter  IntegratorICVariant=Disabled  ExternalResetVariant=Disabled  TRSumVariant=Passthrough  SumFdbkVariant=Disabled  SumVariant=Sum_PD  TsampFilterVariant=InternalTs  TsampNgainVariant=Passthrough  TsampIntegralVariant=Disabled_SignalSpec  ExternalSaturationOutDataTypeStr=Inherit: Same as second input
  PID Controller2 : slpidlib/PID Controller  Controller=I  Form=Parallel  TimeDomain=Discrete-time  UseExternalTs=off  SampleTime=-1  IntegratorMethod=Forward Euler  FilterMethod=Forward Euler  ControllerParametersSource=internal  P=0  I=1  D=1  UseFilter=on  N=100  TunerSelectOption=Transfer Function Based (PID Tuner App)  InitialConditionSource=internal  InitialConditionForIntegrator=0  InitialConditionForFilter=0  DifferentiatorICPrevScaledInput=0  ExternalReset=none  TrackingMode=off  Kt=1  LimitOutput=off  SatLimitsSource=internal  UpperSaturationLimit=inf  LowerSaturationLimit=-inf  LinearizeAsGain=on  AntiWindupMode=none  Kb=1  POutMin=[]  POutMax=[]  IOutMin=[]  IOutMax=[]  DOutMin=[]  DOutMax=[]  NOutMin=[]  NOutMax=[]  SumOutMin=[]  SumOutMax=[]  SaturationOutMin=[]  SaturationOutMax=[]  PParamMin=[]  PParamMax=[]  IParamMin=[]  IParamMax=[]  DParamMin=[]  DParamMax=[]  NParamMin=[]  NParamMax=[]  KbParamMin=[]  KbParamMax=[]  KtParamMin=[]  KtParamMax=[]  KbOutMin=[]  KbOutMax=[]  KtOutMin=[]  KtOutMax=[]  IntegratorOutMin=[]  IntegratorOutMax=[]  FilterOutMin=[]  FilterOutMax=[]  SumI1OutMin=[]  SumI1OutMax=[]  SumI2OutMin=[]  SumI2OutMax=[]  SumI3OutMin=[]  SumI3OutMax=[]  SumI4OutMin=[]  SumI4OutMax=[]  SumDOutMin=[]  SumDOutMax=[]  DifferentiatorOutMin=[]  DifferentiatorOutMax=[]  FilterDiffOutCoefMin=[]  FilterDiffOutCoefMax=[]  ReciprocalOutMin=[]  ReciprocalOutMax=[]  SumDenOutMin=[]  SumDenOutMax=[]  SumNumOutMin=[]  SumNumOutMax=[]  DivideOutMin=[]  DivideOutMax=[]  UdiffTsProdOutMin=[]  UdiffTsProdOutMax=[]  NTsProdOutMin=[]  NTsProdOutMax=[]  UintegralTsProdOutMin=[]  UintegralTsProdOutMax=[]  UngainTsProdOutMin=[]  UngainTsProdOutMax=[]  IntegratorContinuousStateAttributes=''  IntegratorStateMustResolveToSignalObject=off  IntegratorRTWStateStorageClass=Auto  FilterContinuousStateAttributes=''  FilterStateMustResolveToSignalObject=off  FilterRTWStateStorageClass=Auto  ParallelPVariant=Disabled  IdealPVariant=Disabled  IVariant=InternalParameters  DVariant=Disabled  IntegratorVariant=Discrete  SatVariant=Disabled  AWVariant=Passthrough  PCopyVariant=Disabled  TRVariant=Disabled  FdbkBlocksVariant=Forward  IdealPFdbkVariant=Disabled  SatFdbkVariant=Disabled  DerivativeFilterVariant=Disabled  NVariant=Disabled  NCopyVariant=Disabled_SignalSpec  FilterICVariant=Disabled  IntegratorICVariant=InternalICs  ExternalResetVariant=Disabled  TRSumVariant=Passthrough  SumFdbkVariant=Disabled  SumVariant=Passthrough_I  TsampFilterVariant=InternalTs  TsampNgainVariant=Passthrough  TsampIntegralVariant=Passthrough  ExternalSaturationOutDataTypeStr=Inherit: Same as second input
  Sum : Sum  Inputs=|+-
  Ie : Outport
  dr : Outport  Port=2
  dy : Outport  Port=3
  wires:
  PID Controller/1 -> dr/1
  PID Controller1/1 -> dy/1
  y/1 -> Sum/2, PID Controller1/1
  r/1 -> PID Controller/1, Sum/1
  Sum/1 -> PID Controller2/1
  PID Controller2/1 -> Ie/1

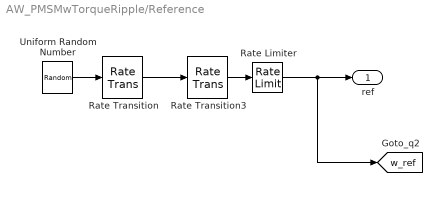
== system AW_PMSMwTorqueRipple/Reference ==
  Rate Limiter : RateLimiter  RisingSlewLimit=0.2/0.1  FallingSlewLimit=-0.2/0.1  SampleTimeMode=inherited
  Rate Transition : RateTransition  InitialCondition=0.05
  Rate Transition3 : RateTransition  OutPortSampleTime=ts
  Uniform Random Number : UniformRandomNumber  Minimum=-2  Maximum=2  Seed=123  SampleTime=50.0
  ref : Outport  VectorParamsAs1DForOutWhenUnconnected=off
  tag scope: w_ref=global
  wires:
  Rate Transition/1 -> Rate Transition3/1
  Uniform Random Number/1 -> Rate Transition/1
  Rate Transition3/1 -> Rate Limiter/1
  Rate Limiter/1 -> [w_ref], ref/1

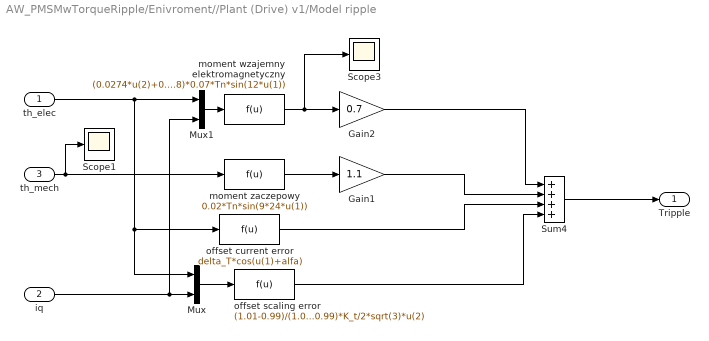
== system AW_PMSMwTorqueRipple/Enivroment//Plant (Drive) v1/Model ripple ==
  th_elec : Inport
  iq : Inport  Port=2
  th_mech : Inport  Port=3
  Gain1 : Gain  Gain=1.1  SaturateOnIntegerOverflow=on  OutDataTypeStr=Inherit: Same as input  ParamDataTypeStr=Inherit: Same as input
  Gain2 : Gain  Gain=0.7  SaturateOnIntegerOverflow=on  OutDataTypeStr=Inherit: Same as input  ParamDataTypeStr=Inherit: Same as input
  Mux : Mux  Inputs=2
  Mux1 : Mux  Inputs=2
  Scope1 : Scope
  Scope3 : Scope
  Sum4 : Sum  Inputs=++++  InputSameDT=on  SaturateOnIntegerOverflow=on  OutDataTypeStr=Inherit: Same as first input
  moment wzajemny elektromagnetyczny : Fcn  Expr=(0.0274*u(2)+0.0438)*Tn*sin(6*u(1))+(0.0274*u(2)+0.0438)*0.07*Tn*sin(12*u(1))
  moment zaczepowy : Fcn  Expr=0.02*Tn*sin(9*24*u(1))
  offset current error : Fcn  Expr=delta_T*cos(u(1)+alfa)
  offset scaling error : Fcn  Expr=(1.01-0.99)/(1.01*0.99)*K_t/sqrt(3)*u[2]*cos(2*u(1)+pi/3)+(1.01-0.99)/(1.01*0.99)*K_t/2*sqrt(3)*u(2)
  Tripple : Outport  VectorParamsAs1DForOutWhenUnconnected=off
  wires:
  moment wzajemny elektromagnetyczny/1 -> Scope3/1, Gain2/1
  Mux/1 -> offset scaling error/1
  th_elec/1 -> offset current error/1, Mux/1, Mux1/1
  iq/1 -> Mux/2, Mux1/2
  Sum4/1 -> Tripple/1
  Mux1/1 -> moment wzajemny elektromagnetyczny/1
  th_mech/1 -> Scope1/1, moment zaczepowy/1
  moment zaczepowy/1 -> Gain1/1
  offset current error/1 -> Sum4/3
  offset scaling error/1 -> Sum4/4
  Gain1/1 -> Sum4/2
  Gain2/1 -> Sum4/1

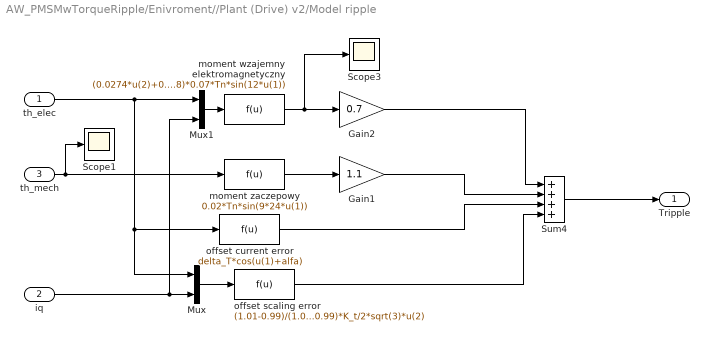
== system AW_PMSMwTorqueRipple/Enivroment//Plant (Drive) v2/Model ripple ==
  th_elec : Inport
  iq : Inport  Port=2
  th_mech : Inport  Port=3
  Gain1 : Gain  Gain=1.1  SaturateOnIntegerOverflow=on  OutDataTypeStr=Inherit: Same as input  ParamDataTypeStr=Inherit: Same as input
  Gain2 : Gain  Gain=0.7  SaturateOnIntegerOverflow=on  OutDataTypeStr=Inherit: Same as input  ParamDataTypeStr=Inherit: Same as input
  Mux : Mux  Inputs=2
  Mux1 : Mux  Inputs=2
  Scope1 : Scope
  Scope3 : Scope
  Sum4 : Sum  Inputs=++++  InputSameDT=on  SaturateOnIntegerOverflow=on  OutDataTypeStr=Inherit: Same as first input
  moment wzajemny elektromagnetyczny : Fcn  Expr=(0.0274*u(2)+0.0438)*Tn*sin(6*u(1))+(0.0274*u(2)+0.0438)*0.07*Tn*sin(12*u(1))
  moment zaczepowy : Fcn  Expr=0.02*Tn*sin(9*24*u(1))
  offset current error : Fcn  Expr=delta_T*cos(u(1)+alfa)
  offset scaling error : Fcn  Expr=(1.01-0.99)/(1.01*0.99)*K_t/sqrt(3)*u[2]*cos(2*u(1)+pi/3)+(1.01-0.99)/(1.01*0.99)*K_t/2*sqrt(3)*u(2)
  Tripple : Outport  VectorParamsAs1DForOutWhenUnconnected=off
  wires:
  moment wzajemny elektromagnetyczny/1 -> Scope3/1, Gain2/1
  Mux/1 -> offset scaling error/1
  th_elec/1 -> offset current error/1, Mux/1, Mux1/1
  iq/1 -> Mux/2, Mux1/2
  Sum4/1 -> Tripple/1
  Mux1/1 -> moment wzajemny elektromagnetyczny/1
  th_mech/1 -> Scope1/1, moment zaczepowy/1
  moment zaczepowy/1 -> Gain1/1
  offset current error/1 -> Sum4/3
  offset scaling error/1 -> Sum4/4
  Gain1/1 -> Sum4/2
  Gain2/1 -> Sum4/1

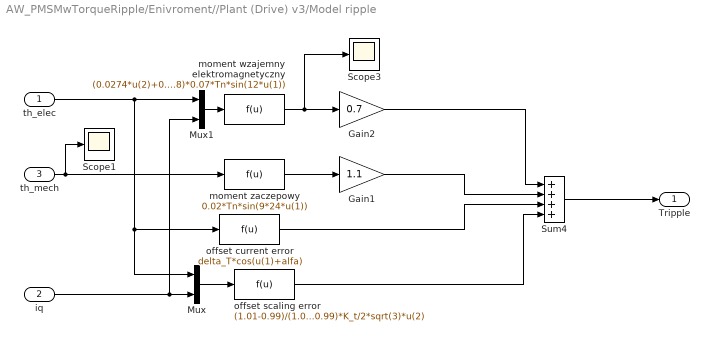
== system AW_PMSMwTorqueRipple/Enivroment//Plant (Drive) v3/Model ripple ==
  th_elec : Inport
  iq : Inport  Port=2
  th_mech : Inport  Port=3
  Gain1 : Gain  Gain=1.1  SaturateOnIntegerOverflow=on  OutDataTypeStr=Inherit: Same as input  ParamDataTypeStr=Inherit: Same as input
  Gain2 : Gain  Gain=0.7  SaturateOnIntegerOverflow=on  OutDataTypeStr=Inherit: Same as input  ParamDataTypeStr=Inherit: Same as input
  Mux : Mux  Inputs=2
  Mux1 : Mux  Inputs=2
  Scope1 : Scope
  Scope3 : Scope
  Sum4 : Sum  Inputs=++++  InputSameDT=on  SaturateOnIntegerOverflow=on  OutDataTypeStr=Inherit: Same as first input
  moment wzajemny elektromagnetyczny : Fcn  Expr=(0.0274*u(2)+0.0438)*Tn*sin(6*u(1))+(0.0274*u(2)+0.0438)*0.07*Tn*sin(12*u(1))
  moment zaczepowy : Fcn  Expr=0.02*Tn*sin(9*24*u(1))
  offset current error : Fcn  Expr=delta_T*cos(u(1)+alfa)
  offset scaling error : Fcn  Expr=(1.01-0.99)/(1.01*0.99)*K_t/sqrt(3)*u[2]*cos(2*u(1)+pi/3)+(1.01-0.99)/(1.01*0.99)*K_t/2*sqrt(3)*u(2)
  Tripple : Outport  VectorParamsAs1DForOutWhenUnconnected=off
  wires:
  moment wzajemny elektromagnetyczny/1 -> Scope3/1, Gain2/1
  Mux/1 -> offset scaling error/1
  th_elec/1 -> offset current error/1, Mux/1, Mux1/1
  iq/1 -> Mux/2, Mux1/2
  Sum4/1 -> Tripple/1
  Mux1/1 -> moment wzajemny elektromagnetyczny/1
  th_mech/1 -> Scope1/1, moment zaczepowy/1
  moment zaczepowy/1 -> Gain1/1
  offset current error/1 -> Sum4/3
  offset scaling error/1 -> Sum4/4
  Gain1/1 -> Sum4/2
  Gain2/1 -> Sum4/1

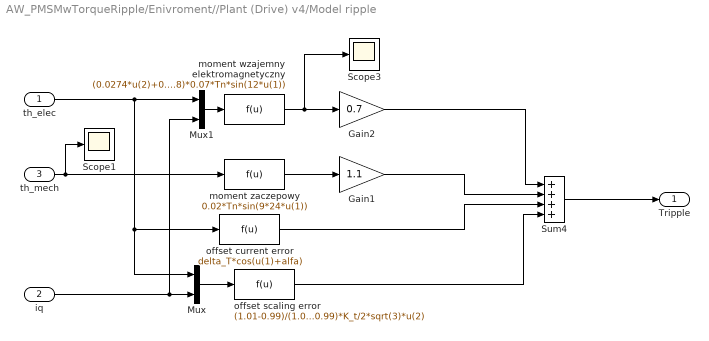
== system AW_PMSMwTorqueRipple/Enivroment//Plant (Drive) v4/Model ripple ==
  th_elec : Inport
  iq : Inport  Port=2
  th_mech : Inport  Port=3
  Gain1 : Gain  Gain=1.1  SaturateOnIntegerOverflow=on  OutDataTypeStr=Inherit: Same as input  ParamDataTypeStr=Inherit: Same as input
  Gain2 : Gain  Gain=0.7  SaturateOnIntegerOverflow=on  OutDataTypeStr=Inherit: Same as input  ParamDataTypeStr=Inherit: Same as input
  Mux : Mux  Inputs=2
  Mux1 : Mux  Inputs=2
  Scope1 : Scope
  Scope3 : Scope
  Sum4 : Sum  Inputs=++++  InputSameDT=on  SaturateOnIntegerOverflow=on  OutDataTypeStr=Inherit: Same as first input
  moment wzajemny elektromagnetyczny : Fcn  Expr=(0.0274*u(2)+0.0438)*Tn*sin(6*u(1))+(0.0274*u(2)+0.0438)*0.07*Tn*sin(12*u(1))
  moment zaczepowy : Fcn  Expr=0.02*Tn*sin(9*24*u(1))
  offset current error : Fcn  Expr=delta_T*cos(u(1)+alfa)
  offset scaling error : Fcn  Expr=(1.01-0.99)/(1.01*0.99)*K_t/sqrt(3)*u[2]*cos(2*u(1)+pi/3)+(1.01-0.99)/(1.01*0.99)*K_t/2*sqrt(3)*u(2)
  Tripple : Outport  VectorParamsAs1DForOutWhenUnconnected=off
  wires:
  moment wzajemny elektromagnetyczny/1 -> Scope3/1, Gain2/1
  Mux/1 -> offset scaling error/1
  th_elec/1 -> offset current error/1, Mux/1, Mux1/1
  iq/1 -> Mux/2, Mux1/2
  Sum4/1 -> Tripple/1
  Mux1/1 -> moment wzajemny elektromagnetyczny/1
  th_mech/1 -> Scope1/1, moment zaczepowy/1
  moment zaczepowy/1 -> Gain1/1
  offset current error/1 -> Sum4/3
  offset scaling error/1 -> Sum4/4
  Gain1/1 -> Sum4/2
  Gain2/1 -> Sum4/1
